simulink model "CommandePID"  (R2017a)
settings: Solver=VariableStepAuto  StartTime=0.0  StopTime=10  RelTol=1e-3
libraries: simulink x1
settings Model: Creator=PC  LastModifiedBy=PC

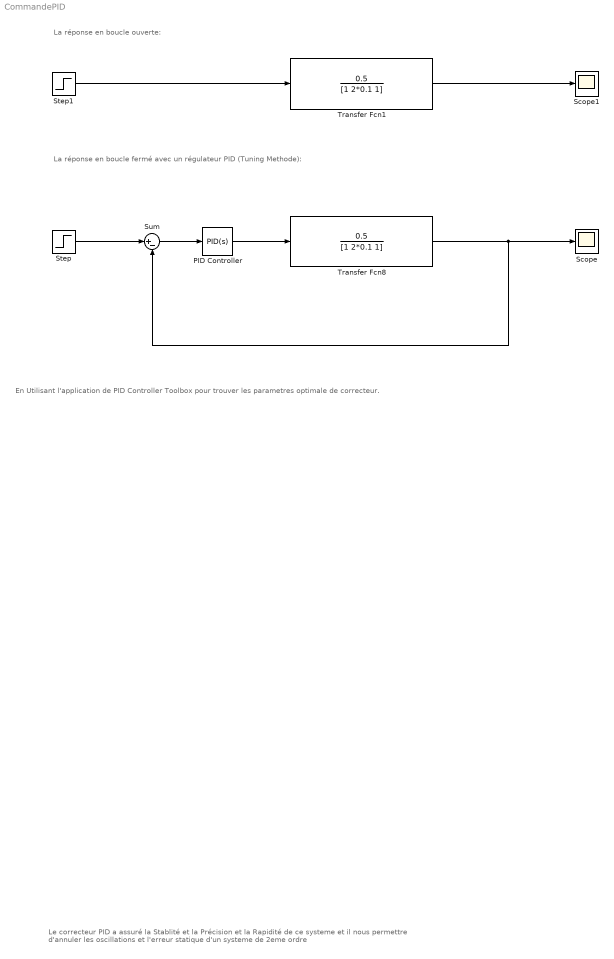
== system CommandePID ==
  note: Le correcteur PID a assuré la Stablité et la Précision et la Rapidité de ce systeme
      | et il nous permettre d'annuler les oscillations et l'erreur statique d'un systeme de 2eme ordre
  note: La réponse en boucle ouverte:
  note: La réponse en boucle fermé avec un régulateur PID (Tuning Methode):
  note: En Utilisant l'application de PID Controller Toolbox pour trouver les parametres optimale de correcteur.
  PID Controller : simulink/Continuous/PID Controller  Controller=PID  TimeDomain=Continuous-time  SampleTime=-1  IntegratorMethod=Forward Euler  FilterMethod=Forward Euler  Form=Parallel  UseFilter=on  ControllerParametersSource=internal  P=140.387916085064  I=124.22778960369  D=39.099622895094  N=209.794311620465  InitialConditionSource=internal  InitialConditionForIntegrator=0  InitialConditionForFilter=0  ExternalReset=none  LimitOutput=off  UpperSaturationLimit=inf  LowerSaturationLimit=-inf  LinearizeAsGain=on  AntiWindupMode=none  Kb=1  TrackingMode=off  Kt=1  PParamMin=[]  PParamMax=[]  IParamMin=[]  IParamMax=[]  DParamMin=[]  DParamMax=[]  NParamMin=[]  NParamMax=[]  KbParamMin=[]  KbParamMax=[]  KtParamMin=[]  KtParamMax=[]  POutMin=[]  POutMax=[]  IOutMin=[]  IOutMax=[]  DOutMin=[]  DOutMax=[]  NOutMin=[]  NOutMax=[]  KbOutMin=[]  KbOutMax=[]  KtOutMin=[]  KtOutMax=[]  IntegratorOutMin=[]  IntegratorOutMax=[]  FilterOutMin=[]  FilterOutMax=[]  SumOutMin=[]  SumOutMax=[]  SumI1OutMin=[]  SumI1OutMax=[]  SumI2OutMin=[]  SumI2OutMax=[]  SumI3OutMin=[]  SumI3OutMax=[]  SumDOutMin=[]  SumDOutMax=[]  SaturationOutMin=[]  SaturationOutMax=[]  IntegratorContinuousStateAttributes=''  IntegratorStateMustResolveToSignalObject=off  IntegratorRTWStateStorageClass=Auto  FilterContinuousStateAttributes=''  FilterStateMustResolveToSignalObject=off  FilterRTWStateStorageClass=Auto  DifferentiatorICPrevScaledInput=0  DifferentiatorOutMin=[]  DifferentiatorOutMax=[]  InitialConditionSetting=State (most efficient)
  Scope : Scope
  Scope1 : Scope
  Step : Step  Time=0  SampleTime=0
  Step1 : Step  Time=0  SampleTime=0
  Sum : Sum  Inputs=|+-
  Transfer Fcn1 : TransferFcn  Numerator=[0.5]  Denominator=[1 2*0.1 1]
  Transfer Fcn8 : TransferFcn  Numerator=[0.5]  Denominator=[1 2*0.1 1]
  wires:
  Sum/1 -> PID Controller/1
  Step/1 -> Sum/1
  PID Controller/1 -> Transfer Fcn8/1
  Transfer Fcn8/1 -> Sum/2, Scope/1
  Step1/1 -> Transfer Fcn1/1
  Transfer Fcn1/1 -> Scope1/1
